simulink model "FOC"  (R2015b)
settings: Solver=ode4  StartTime=0.0  StopTime=10.0  FixedStep=1e-3  RelTol=1e-3
settings Model: Creator=E27269  LastModifiedBy=e27269
settings DataIOCC: SaveFormat=Array
settings DebuggingCC: SolverPrmCheckMsg=warning
settings HardwareCC: ProdBitPerPointer=32  ProdLargestAtomicFloat=None  ProdIntDivRoundTo=Undefined  ProdEndianess=Unspecified  ProdWordSize=32  ProdHWDeviceType=32-bit Generic
settings GRTTargetCC: GeneratePreprocessorConditionals=Disable all
settings ConfigComp: CovModelRefEnable=Off  CovSFcnEnable=off

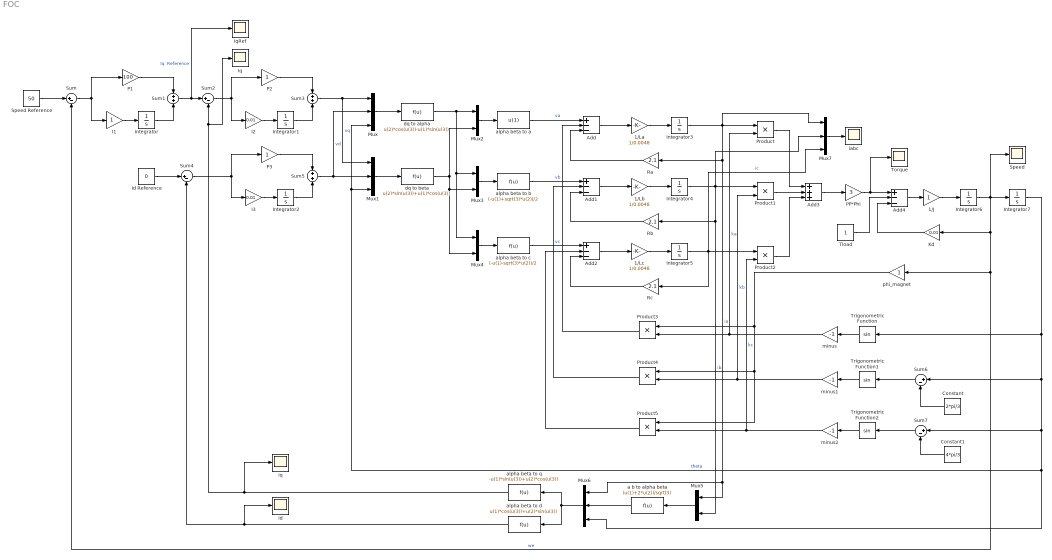
== system FOC ==
  1/J : Gain
  1/La : Gain  Gain=1/0.0048
  1/Lb : Gain  Gain=1/0.0048
  1/Lc : Gain  Gain=1/0.0048
  Add{,1..2,4} (4 alike) : Sum  Inputs=+--
  Add3 : Sum  Inputs=+++
  Constant : Constant  Value=2*pi/3
  Constant1 : Constant  Value=4*pi/3
  I1 : Gain
  I2 : Gain  Gain=0.01
  I3 : Gain  Gain=0.01
  Id Reference : Constant  Value=0
  Integrator{,1..7} (8 alike) : Integrator
  Iq : Scope
  IqRef : Scope
  Kd : Gain  Gain=0.01
  Mux{,1,6..7} (4 alike) : Mux  Inputs=3
  Mux{2..5} (4 alike) : Mux  Inputs=2
  P1 : Gain  Gain=100
  P2 : Gain
  P3 : Gain
  PP*Phi : Gain  Gain=3
  Product{,1..5} (6 alike) : Product
  Ra : Gain  Gain=2.1
  Rb : Gain  Gain=2.1
  Rc : Gain  Gain=2.1
  Speed : Scope
  Speed Reference : Constant  Value=50
  Sum{,2,4,6..7} (5 alike) : Sum  Inputs=|+-
  Sum1 : Sum  Inputs=+|+
  Sum3 : Sum  Inputs=+|+
  Sum5 : Sum  Inputs=+|+
  Tload : Constant
  Torque : Scope
  Trigonometric Function : Trigonometry
  Trigonometric Function1 : Trigonometry
  Trigonometric Function2 : Trigonometry
  a b to alpha beta : Fcn  Expr=(u(1)+2*u(2))/sqrt(3)
  alpha beta to a : Fcn  Expr=u(1)
  alpha beta to b : Fcn  Expr=(-u(1)+sqrt(3)*u(2))/2
  alpha beta to c : Fcn  Expr=(-u(1)-sqrt(3)*u(2))/2
  alpha beta to d : Fcn  Expr=u(1)*cos(u(3))+u(2)*sin(u(3))
  alpha beta to q : Fcn  Expr=-u(1)*sin(u(3))+u(2)*cos(u(3))
  dq to alpha : Fcn  Expr=u(2)*cos(u(3))-u(1)*sin(u(3))
  dq to beta : Fcn  Expr=u(2)*sin(u(3))+u(1)*cos(u(3))
  iabc : Scope
  id : Scope
  iq : Scope
  minus : Gain  Gain=-1
  minus1 : Gain  Gain=-1
  minus2 : Gain  Gain=-1
  phi_magnet : Gain
  wires:
  Speed Reference/1 -> Sum/1
  I1/1 -> Integrator/1
  Sum/1 -> I1/1, P1/1
  P1/1 -> Sum1/1
  Integrator/1 -> Sum1/2
  Sum1/1 -> IqRef/1, Sum2/1  "Iq  Reference"
  I2/1 -> Integrator1/1
  Sum2/1 -> P2/1, I2/1
  P2/1 -> Sum3/1
  Integrator1/1 -> Sum3/2
  Sum3/1 -> Mux/1, Mux1/1  "vq"
  Id Reference/1 -> Sum4/1
  I3/1 -> Integrator2/1
  Sum4/1 -> I3/1, P3/1
  P3/1 -> Sum5/1
  Integrator2/1 -> Sum5/2
  Sum5/1 -> Mux1/2, Mux/2  "vd"
  Mux/1 -> dq to alpha/1
  Mux1/1 -> dq to beta/1
  dq to alpha/1 -> Mux3/1, Mux4/1, Mux2/1
  dq to beta/1 -> Mux3/2, Mux4/2, Mux2/2
  Mux2/1 -> alpha beta to a/1
  Mux3/1 -> alpha beta to b/1
  Mux4/1 -> alpha beta to c/1
  alpha beta to a/1 -> Add/1  "va"
  1/La/1 -> Integrator3/1
  Integrator3/1 -> Mux7/1, Product/1, Mux6/1, Mux5/1, Ra/1  "ia"
  Add/1 -> 1/La/1
  Ra/1 -> Add/3
  alpha beta to b/1 -> Add1/1  "vb"
  1/Lb/1 -> Integrator4/1
  Add1/1 -> 1/Lb/1
  Rb/1 -> Add1/3
  alpha beta to c/1 -> Add2/1  "vc"
  1/Lc/1 -> Integrator5/1
  Integrator5/1 -> Mux7/3, Product2/1, Rc/1  "ic"
  Add2/1 -> 1/Lc/1
  Rc/1 -> Add2/3
  Integrator4/1 -> Mux7/2, Product1/1, Mux5/2, Rb/1  "ib"
  Product/1 -> Add3/1
  Product1/1 -> Add3/2
  Product2/1 -> Add3/3
  Add3/1 -> PP*Phi/1
  PP*Phi/1 -> Torque/1, Add4/1
  Add4/1 -> 1/J/1
  1/J/1 -> Integrator6/1
  Integrator6/1 -> Speed/1, phi_magnet/1, Sum/2, Kd/1, Integrator7/1  "we"
  Kd/1 -> Add4/3
  Tload/1 -> Add4/2
  Integrator7/1 -> Trigonometric Function/1, Sum6/1, Mux6/3, Mux1/3, Mux/3, Sum7/1  "theta"
  Trigonometric Function/1 -> minus/1
  phi_magnet/1 -> Product3/1, Product4/1, Product5/1
  Product3/1 -> Add/2
  Sum6/1 -> Trigonometric Function1/1
  Sum7/1 -> Trigonometric Function2/1
  Constant/1 -> Sum6/2
  Constant1/1 -> Sum7/2
  Trigonometric Function1/1 -> minus1/1
  Trigonometric Function2/1 -> minus2/1
  Product4/1 -> Add1/2
  Product5/1 -> Add2/2
  Mux5/1 -> a b to alpha beta/1
  a b to alpha beta/1 -> Mux6/2
  Mux6/1 -> alpha beta to d/1, alpha beta to q/1
  alpha beta to d/1 -> id/1, Sum4/2
  Mux7/1 -> iabc/1
  minus/1 -> Product3/2, Product/2  "ka"
  minus1/1 -> Product1/2, Product4/2  "kb"
  minus2/1 -> Product2/2, Product5/2  "kc"
  alpha beta to q/1 -> iq/1, Iq/1, Sum2/2
